simulink model "project_raspberry"  (R2024a)
settings: Solver=FixedStepAuto  StartTime=0.0  StopTime=inf  RelTol=1e-3  EnableMultiTasking=on
libraries: raspberrypiBasiclib x2, raspberrypiCommlib x2
settings Model: Creator=hp  LastModifiedBy=hp
settings SolverCC: PositivePriorityOrder=on
settings OptimizationCC: EnhancedBackFolding=on  PassReuseOutputArgsAs=Individual arguments  ZeroExternalMemoryAtStartup=off  ZeroInternalMemoryAtStartup=off  MaxStackSize=64  OptimizeBlockOrder=speed  DifferentSizesBufferReuse=on  OptimizationCustomize=off  EfficientTunableParamExpr=on
settings DebuggingCC: ParameterTunabilityLossMsg=error
settings HardwareCC: ProdBitPerPointer=32  ProdBitPerSizeT=32  ProdBitPerPtrDiffT=32  ProdLargestAtomicInteger=Long  ProdLargestAtomicFloat=Double  ProdWordSize=32  ProdLongLongMode=on  ProdHWDeviceType=ARM Compatible->ARM Cortex  UseEmbeddedCoderFeatures=off  UseSimulinkCoderFeatures=off
settings RTWCC: Description=Embedded Coder  SystemTargetFile=ert.tlc  HardwareBoard=Raspberry Pi  TLCOptions="-aInlineSetEventsForThisBaseRateFcn=TLC_FALSE -aSuppressMultiTaskScheduler=TLC_FALSE  -aRateBasedStepFcn=0"  TemplateMakefile=ert_default_tmf  Toolchain=GNU GCC Embedded Linux  BuildConfiguration=Faster Runs
settings CodeAppCC: ForceParamTrailComments=on  IgnoreCustomStorageClasses=off  OperatorAnnotations=on  SimulinkDataObjDesc=on  SFDataObjDesc=on  InsertBlockDesc=on
settings ERTTargetCC: SupportNonInlinedSFcns=on  SupportVariableSizeSignals=on  ExtModeTransport=2  ExtModeStaticAlloc=on  ExtModeMexFile=ext_xcp  ExtModeIntrfLevel=Level2 - Open

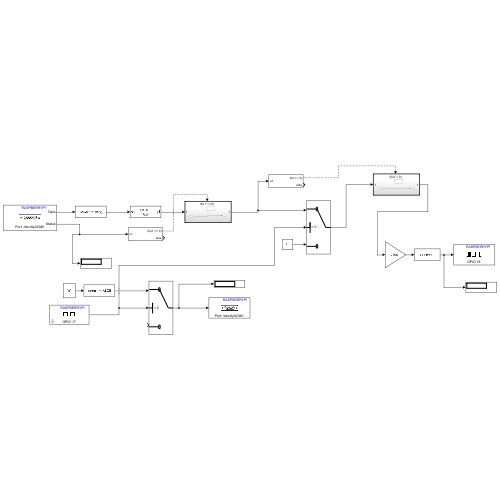
[thumbnail: Simulink's stored preview of the top-level diagram]
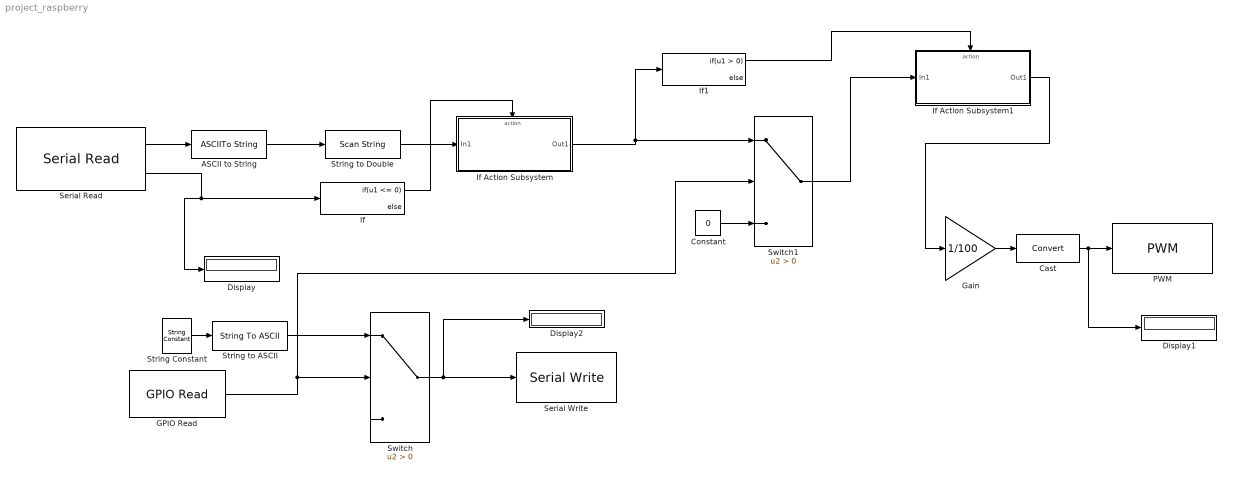
== system project_raspberry ==
  ASCII to String : ASCIIToString
  Cast : DataTypeConversion  SaturateOnIntegerOverflow=off  RndMeth=Floor
  Constant : Constant  Value=0
  Display : Display
  Display1 : Display
  Display2 : Display
  GPIO Read : raspberrypiBasiclib/GPIO Read  board=Pi 3 Model B+  gpio=17  internalResistor=Off  sampleTime=0.1  direction=Input  blockPlatform=Raspberry Pi
  Gain : Gain  Gain=1/100
  If : If  IfExpression=u1 <= 0
  If Action Subsystem : Subsystem  TreatAsAtomicUnit=on
  If Action Subsystem1 : Subsystem  TreatAsAtomicUnit=on
  If1 : If
  PWM : raspberrypiBasiclib/PWM  board=Pi 3 Model B+  Pin_=18  Frequency=500  blockPlatform=Raspberry Pi
  Serial Read : raspberrypiCommlib/Serial Read  board=Pi 3 Model B  SCIModule_=/dev/ttyACM0  Baudrate_=115200  Parity=None  StopBits_=1  HardwareFlowControl=None  ByteOrder=LittleEndian  DataLength=2  DataType=uint8  OutputStatus=on  SampleTime=0.1  blockPlatform=RaspberryPi
  Serial Write : raspberrypiCommlib/Serial Write  board=Pi 3 Model B+  SCIModule_=/dev/ttyACM0  Baudrate_=115200  Parity=None  StopBits_=1  HardwareFlowControl=None  ByteOrder=LittleEndian  OutputStatus=off  blockPlatform=RaspberryPi
  String Constant : StringConstant  String="\"a\""
  String to ASCII : StringToASCII
  String to Double : ScanString  Format="\"%d\""
  Switch : Switch  Criteria=u2 > Threshold  SaturateOnIntegerOverflow=off  InputSameDT=off
  Switch1 : Switch  Criteria=u2 > Threshold  SaturateOnIntegerOverflow=off  InputSameDT=off
  wires:
  String Constant/1 -> String to ASCII/1
  Switch/1 -> Display2/1, Serial Write/1
  Serial Read/2 -> If/1, Display/1
  ASCII to String/1 -> String to Double/1
  Serial Read/1 -> ASCII to String/1
  If/1 -> If Action Subsystem/Action
  String to Double/1 -> If Action Subsystem/1(In1)
  String to ASCII/1 -> Switch/1
  GPIO Read/1 -> Switch/2, Switch1/2
  Constant/1 -> Switch1/3
  Gain/1 -> Cast/1
  Cast/1 -> PWM/1, Display1/1
  If Action Subsystem/1(Out1) -> If1/1, Switch1/1
  If1/1 -> If Action Subsystem1/Action
  Switch1/1 -> If Action Subsystem1/1(In1)
  If Action Subsystem1/1(Out1) -> Gain/1

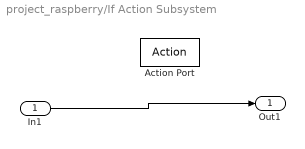
== system project_raspberry/If Action Subsystem ==
  In1 : Inport
  Action Port : ActionPort  ActionPortLabel=if(u1 <= 0)
  Out1 : Outport
  wires:
  In1/1 -> Out1/1

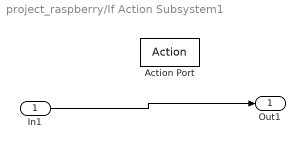
== system project_raspberry/If Action Subsystem1 ==
  In1 : Inport
  Action Port : ActionPort  ActionPortLabel=if(u1 > 0)
  Out1 : Outport
  wires:
  In1/1 -> Out1/1
